simulink subsystem "rss_RefVltgLimCalc"  (R2023a)
settings: Solver=VariableStepAuto  StartTime=0.0  StopTime=10.0  RelTol=1e-3
undefined symbols (not defined in the file): Cdbl_uPhVltgMaxVal, Cdbl_uSplyVltgMaxVal, Gu16_rMaxVltgAmpRat_C
libraries: lib_conversion x1, lib_right_angle_side_length_calculator x1
settings Model: Creator=xiaoqiang.yuan  LastModifiedBy=xiaoqiang.yuan

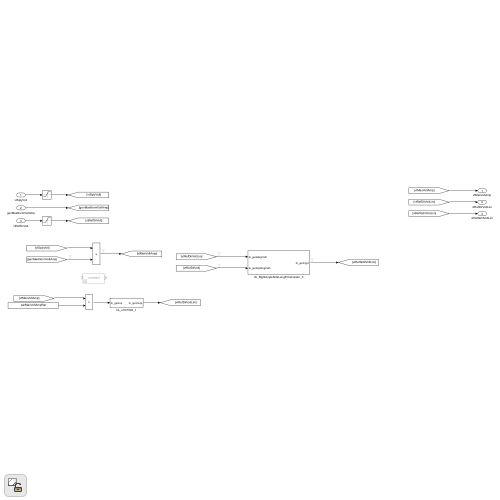
[thumbnail: Simulink's stored preview of the top-level diagram]
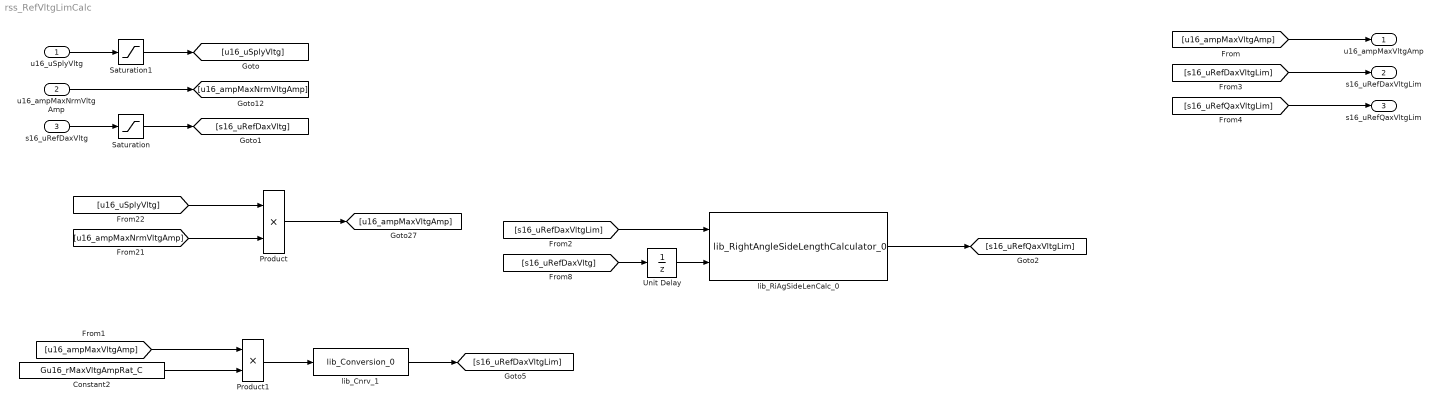
== system rss_RefVltgLimCalc ==
  u16_uSplyVltg : Inport  OutDataTypeStr=dt_Standardize_u16p15b0
  u16_ampMaxNrmVltgAmp : Inport  Port=2  OutDataTypeStr=dt_DutyCycl_u16p15b0
  s16_uRefDaxVltg : Inport  Port=3  OutDataTypeStr=dt_Standardize_s16p15b0
  Constant2 : Constant  Value=Gu16_rMaxVltgAmpRat_C
  Product : Product  RndMeth=Simplest  OutDataTypeStr=Inherit: Same as first input
  Product1 : Product  OutDataTypeStr=Inherit: Inherit via back propagation
  Saturation : Saturate  UpperLimit=Cdbl_uPhVltgMaxVal  LowerLimit=-Cdbl_uPhVltgMaxVal
  Saturation1 : Saturate  UpperLimit=Cdbl_uSplyVltgMaxVal  LowerLimit=0
  Unit Delay : UnitDelay  SampleTime=-1  HasFrameUpgradeWarning=on
  lib_Cnrv_1 : lib_conversion/lib_Conversion_0  lb_parDataType=dt_Standardize_s16p15b0  lb_parOutpMaxVal=[]  lb_parOutpMinVal=[]  lb_parSatFlag=off
  lib_RiAgSideLenCalc_0 : lib_right_angle_side_length_calculator/lib_RightAngleSideLengthCalculator_0  lb_parLktSize=512  lb_parOutpDataType=dt_Standardize_s16p15b0
  u16_ampMaxVltgAmp : Outport  OutDataTypeStr=dt_Standardize_u16p15b0
  s16_uRefDaxVltgLim : Outport  Port=2  OutDataTypeStr=dt_Standardize_s16p15b0
  s16_uRefQaxVltgLim : Outport  Port=3  OutDataTypeStr=dt_Standardize_s16p15b0
  wires:
  [u16_uSplyVltg] -> Product/1
  [u16_ampMaxVltgAmp] -> Product1/1
  [u16_ampMaxNrmVltgAmp] -> Product/2
  Product/1 -> [u16_ampMaxVltgAmp]
  Saturation1/1 -> [u16_uSplyVltg]
  u16_uSplyVltg/1 -> Saturation1/1
  u16_ampMaxNrmVltgAmp/1 -> [u16_ampMaxNrmVltgAmp]
  Saturation/1 -> [s16_uRefDaxVltg]
  s16_uRefDaxVltg/1 -> Saturation/1
  [u16_ampMaxVltgAmp] -> u16_ampMaxVltgAmp/1
  [s16_uRefDaxVltg] -> Unit Delay/1
  [s16_uRefDaxVltgLim] -> lib_RiAgSideLenCalc_0/1
  [s16_uRefDaxVltgLim] -> s16_uRefDaxVltgLim/1
  lib_RiAgSideLenCalc_0/1 -> [s16_uRefQaxVltgLim]
  [s16_uRefQaxVltgLim] -> s16_uRefQaxVltgLim/1
  Product1/1 -> lib_Cnrv_1/1
  Constant2/1 -> Product1/2
  lib_Cnrv_1/1 -> [s16_uRefDaxVltgLim]
  Unit Delay/1 -> lib_RiAgSideLenCalc_0/2
